simulink model "harm_comp"  (R2020a)
settings: Solver=VariableStepAuto  StartTime=0.0  StopTime=10.0  RelTol=1e-3
values from neighbouring files (symbols this model uses):
  B13 = -params.lmda_f_dc    [run_harmonic_compensation.m]
  comp_table1 = [comp_table1; real(vecs(1,:)*diag(vals)*inv_vecs)]    [run_harmonic_compensation.m]
  Kd0 = [1722.92514708863,-0.149487775533096,     -243.708496078677,0;     0.158174537169950,1528.50661836498,     0,-216.219080907873]    [run_harmonic_compensation.m]
  max_predq = .15    (= 0.15)    [run_harmonic_compensation.m]
  P = params.Poles    [run_harmonic_compensation.m]
  ss_d = H(2,2)    [run_harmonic_compensation.m]
  ss_q = H(1,1)    [run_harmonic_compensation.m]
  start_comp = 50    [run_harmonic_compensation.m]
undefined symbols (not defined in the file or in its folder): baseFreq, T_sw, Vd
settings Model: Creator=adamh  LastModifiedBy=adamh

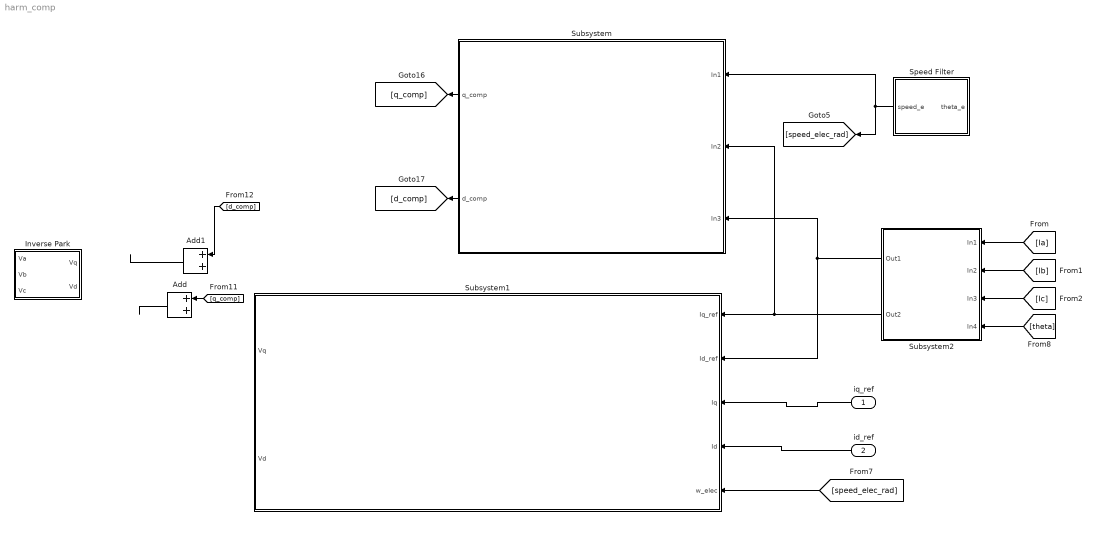
== system harm_comp ==
  iq_ref : Inport
  id_ref : Inport  Port=2
  Add : Sum
  Add1 : Sum
  Inverse Park : Subsystem
  Speed Filter : Subsystem
  Subsystem : Subsystem
      mask Display: image('C:\Users\adamh\Google Drive\AAA Jestie DMD HARMONIC\New_images\Comp_mask.png'); % Use "Edit Image" on toolstrip to change.
  Subsystem1 : Subsystem
      mask Display: image('C:\Users\adamh\Google Drive\AAA Jestie DMD HARMONIC\New_images\Nominal_mask.png'); % Use "Edit Image" on toolstrip to change.
  Subsystem2 : Subsystem
  wires:
  [q_comp] -> Add/1
  [d_comp] -> Add1/1
  Speed Filter/1(speed_e) -> Subsystem/1(In1), [speed_elec_rad]
  Subsystem/1(q_comp) -> [q_comp]
  Subsystem/2(d_comp) -> [d_comp]
  Add1/1 -> ?
  Add/1 -> ?
  iq_ref/1 -> Subsystem1/3("Iq ")
  id_ref/1 -> Subsystem1/4(Id)
  [speed_elec_rad] -> Subsystem1/5(w_elec)
  Subsystem2/2(Out2) -> Subsystem/2(In2), Subsystem1/1(Iq_ref)
  Subsystem2/1(Out1) -> Subsystem1/2(Id_ref), Subsystem/3(In3)
  [Ia] -> Subsystem2/1(In1)
  [Ib] -> Subsystem2/2(In2)
  [Ic] -> Subsystem2/3(In3)
  [theta] -> Subsystem2/4(In4)

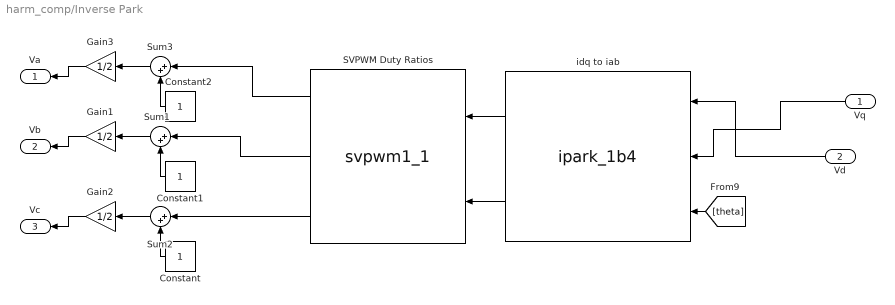
== system harm_comp/Inverse Park ==
  Vq : Inport
  Vd : Inport  Port=2
  Constant : Constant
  Constant1 : Constant
  Constant2 : Constant
  Gain1 : Gain  Gain=1/2
  Gain2 : Gain  Gain=1/2
  Gain3 : Gain  Gain=1/2
  SVPWM Duty Ratios : S-Function  InitFcn=try, set_param(gcb,'FunctionName','svpwm1_1'), end  FunctionName=svpwm1_1  SFunctionModules=svpwm1_1_wrapper  SFunctionDeploymentMode=off  EnableBusSupport=off  mask(S-Function Builder){}
      mask help: Simulink:masks:SFunctionBuilder_MD
      mask init:
      | val = [[.9  0.75 0.75 1 1 .9 .9 1]',[1 1 0.75 0.75 .9 .9 1 .9]'];try , sys = get_param(gcb,'SfunBuilderFcnName');if isempty(sys), sys = get_param(gcb,'FunctionName'); end,catch, sys = get_param(gcb,'FunctionName'); end
      settings: CopyFcn=set_param(gcbh,'LinkStatus','none')  PreSaveFcn=try, set_param(gcb,'FunctionName','svpwm1_1'), end  OpenFcn=sfunctionwizard(gcbh)
      mask Display: plot(val(:,1),val(:,2)),disp(sys), port_label('input',1,'i_alpha'), port_label('input',2,'i_beta'), port_label('output',1,'Ta'), port_label('output',2,'Tb'), port_label('output',3,'Tc')
  Sum1 : Sum  Inputs=|++
  Sum2 : Sum  Inputs=|++
  Sum3 : Sum  Inputs=|++
  idq to iab : S-Function  InitFcn=try, set_param(gcb,'FunctionName','ipark_1b4'), end  FunctionName=ipark_1b4  SFunctionModules=ipark_1b4_wrapper  SFunctionDeploymentMode=off  EnableBusSupport=off  mask(S-Function Builder){}
      mask help: Simulink:masks:SFunctionBuilder_MD
      mask init: same as harm_comp/Inverse Park/SVPWM Duty Ratios
      settings: CopyFcn=set_param(gcbh,'LinkStatus','none')  PreSaveFcn=try, set_param(gcb,'FunctionName','ipark_1b4'), end  OpenFcn=sfunctionwizard(gcbh)
      mask Display: plot(val(:,1),val(:,2)),disp(sys), port_label('input',1,'id'), port_label('input',2,'iq'), port_label('input',3,'theta'), port_label('output',1,'i_alpha'), port_label('output',2,'i_beta')
  Va : Outport
  Vb : Outport  Port=2
  Vc : Outport  Port=3
  wires:
  Sum1/1 -> Gain1/1
  SVPWM Duty Ratios/3 -> Sum2/1
  Sum2/1 -> Gain2/1
  Constant/1 -> Sum2/2
  idq to iab/1 -> SVPWM Duty Ratios/1
  Constant1/1 -> Sum1/2
  SVPWM Duty Ratios/1 -> Sum3/1
  Sum3/1 -> Gain3/1
  idq to iab/2 -> SVPWM Duty Ratios/2
  Gain2/1 -> Vc/1
  [theta] -> idq to iab/3
  SVPWM Duty Ratios/2 -> Sum1/1
  Constant2/1 -> Sum3/2
  Vq/1 -> idq to iab/2
  Vd/1 -> idq to iab/1
  Gain1/1 -> Vb/1
  Gain3/1 -> Va/1

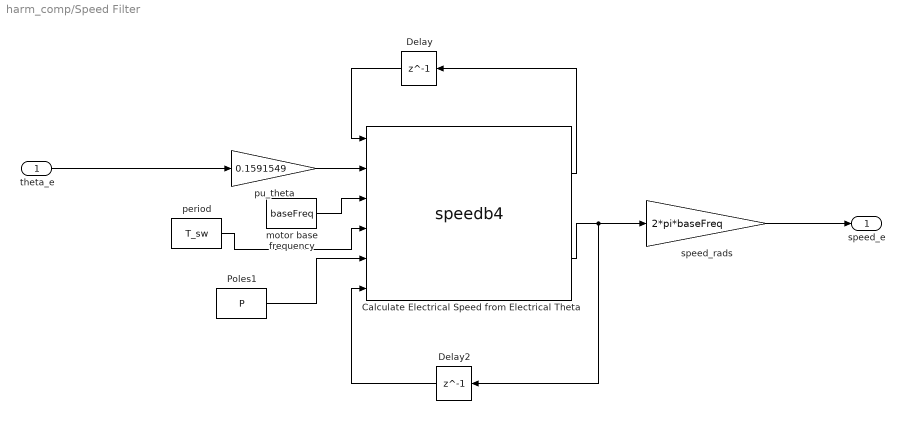
== system harm_comp/Speed Filter ==
  theta_e : Inport
  Calculate Electrical Speed from Electrical Theta : S-Function  InitFcn=try, set_param(gcb,'FunctionName','speedb4'), end  FunctionName=speedb4  SFunctionModules=speedb4_wrapper  SFunctionDeploymentMode=off  EnableBusSupport=off  mask(S-Function Builder){}
      mask help: Simulink:masks:SFunctionBuilder_MD
      mask init: same as harm_comp/Inverse Park/SVPWM Duty Ratios
      settings: CopyFcn=set_param(gcbh,'LinkStatus','none')  PreSaveFcn=try, set_param(gcb,'FunctionName','speedb4'), end  OpenFcn=sfunctionwizard(gcbh)
      mask Display: plot(val(:,1),val(:,2)),disp(sys), port_label('input',1,'oldTheta_in'), port_label('input',2,'theta_in'), port_label('input',3,'baseFreq_in'), port_label('input',4,'T_in'), port_label('input',5,'P_in'), port_label('input',6,'speed_in'), port_label('output',1,'theta_pu'), port_label('output',2,'speed_pu')
  Delay : Delay  DelayLength=1  InitialCondition=0  UseCircularBuffer=on
  Delay2 : Delay  DelayLength=1  InitialCondition=0  UseCircularBuffer=on
  Poles1 : Constant  Value=P
  motor base frequency : Constant  Value=baseFreq
  period : Constant  Value=T_sw
  pu_theta : Gain  Gain=0.1591549
  speed_rads : Gain  Gain=2*pi*baseFreq
  speed_e : Outport
  wires:
  Delay/1 -> Calculate Electrical Speed from Electrical Theta/1
  motor base frequency/1 -> Calculate Electrical Speed from Electrical Theta/3
  Calculate Electrical Speed from Electrical Theta/2 -> speed_rads/1, Delay2/1
  Calculate Electrical Speed from Electrical Theta/1 -> Delay/1
  Poles1/1 -> Calculate Electrical Speed from Electrical Theta/5
  period/1 -> Calculate Electrical Speed from Electrical Theta/4
  pu_theta/1 -> Calculate Electrical Speed from Electrical Theta/2
  Delay2/1 -> Calculate Electrical Speed from Electrical Theta/6
  speed_rads/1 -> speed_e/1
  theta_e/1 -> pu_theta/1

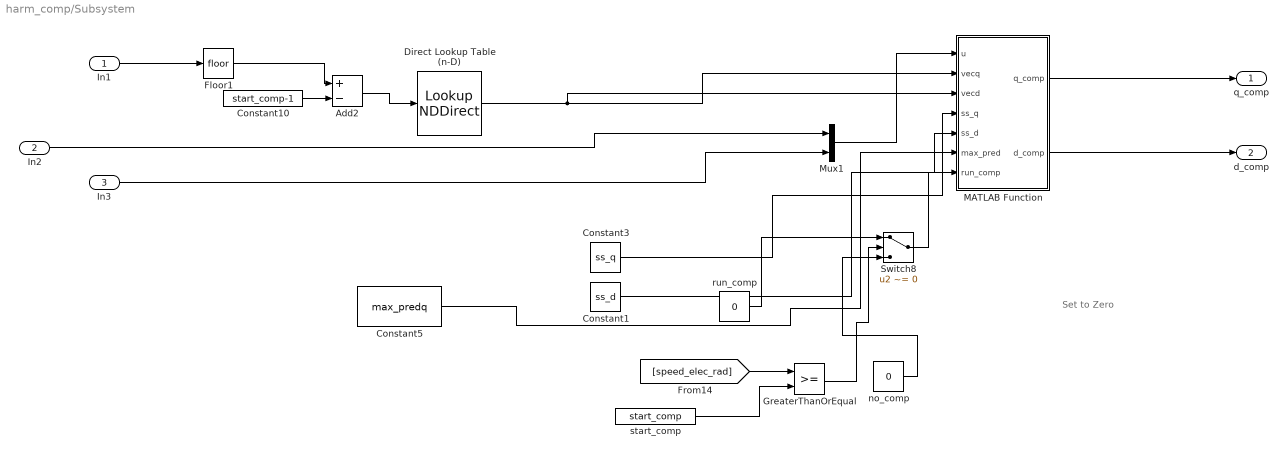
== system harm_comp/Subsystem ==
  note: Set to Zero
  In1 : Inport
  In2 : Inport  Port=2
  In3 : Inport  Port=3
  Add2 : Sum  Inputs=+-
  Constant1 : Constant  Value=ss_d
  Constant10 : Constant  Value=start_comp-1
  Constant3 : Constant  Value=ss_q
  Constant5 : Constant  Value=max_predq
  Direct Lookup Table (n-D) : LookupNDDirect  InputsSelectThisObjectFromTable=Vector  Table=comp_table1'
  Floor1 : Rounding
  GreaterThanOrEqual : RelationalOperator  OutDataTypeStr=boolean  RndMeth=Simplest
  MATLAB Function : MATLAB Function  TreatAsAtomicUnit=on
  Mux1 : Mux  Inputs=2
  Switch8 : Switch  Criteria=u2 ~= 0
  no_comp : Constant  Value=0
  run_comp : Constant  Value=0
  start_comp : Constant  Value=start_comp
  q_comp : Outport
  d_comp : Outport  Port=2
  wires:
  GreaterThanOrEqual/1 -> Switch8/2
  Mux1/1 -> MATLAB Function/1(u)
  no_comp/1 -> Switch8/3
  Constant1/1 -> MATLAB Function/5(ss_d)
  Constant3/1 -> MATLAB Function/4(ss_q)
  Floor1/1 -> Add2/1
  Add2/1 -> Direct Lookup Table (n-D)/1
  Constant5/1 -> MATLAB Function/6(max_pred)
  Direct Lookup Table (n-D)/1 -> MATLAB Function/3(vecd), MATLAB Function/2(vecq)
  start_comp/1 -> GreaterThanOrEqual/2
  [speed_elec_rad] -> GreaterThanOrEqual/1
  Constant10/1 -> Add2/2
  Switch8/1 -> MATLAB Function/7(run_comp)
  run_comp/1 -> Switch8/1
  MATLAB Function/2(d_comp) -> d_comp/1
  In1/1 -> Floor1/1
  MATLAB Function/1(q_comp) -> q_comp/1
  In2/1 -> Mux1/1
  In3/1 -> Mux1/2

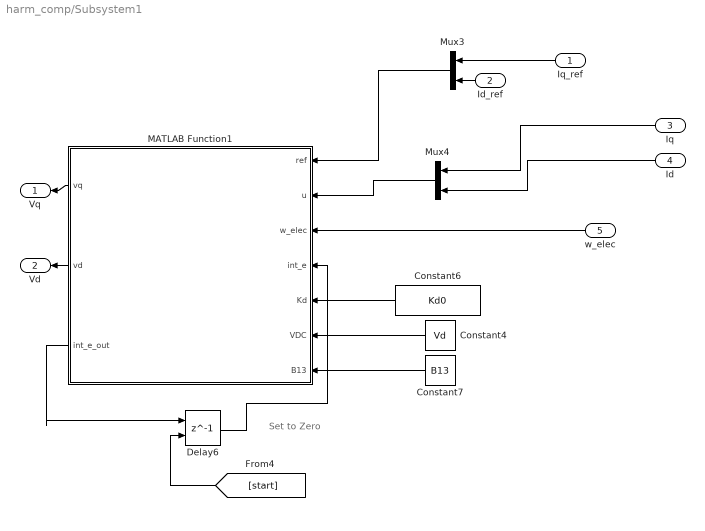
== system harm_comp/Subsystem1 ==
  note: Set to Zero
  Iq_ref : Inport
  Id_ref : Inport  Port=2
  "Iq " : Inport  Port=3
  Id : Inport  Port=4
  w_elec : Inport  Port=5
  Constant4 : Constant  Value=Vd
  Constant6 : Constant  Value=Kd0
  Constant7 : Constant  Value=B13
  Delay6 : Delay  DelayLength=1  ExternalReset=Rising
      settings: InputPortMap=u0,r5
  MATLAB Function1 : MATLAB Function  TreatAsAtomicUnit=on
  Mux3 : Mux  Inputs=2
  Mux4 : Mux  Inputs=2
  Vq : Outport
  Vd : Outport  Port=2
  wires:
  Delay6/1 -> MATLAB Function1/4(int_e)
  MATLAB Function1/3(int_e_out) -> Delay6/1
  Constant7/1 -> MATLAB Function1/7(B13)
  MATLAB Function1/1(vq) -> Vq/1
  Mux4/1 -> MATLAB Function1/2(u)
  Constant4/1 -> MATLAB Function1/6(VDC)
  Mux3/1 -> MATLAB Function1/1(ref)
  Constant6/1 -> MATLAB Function1/5(Kd)
  [start] -> Delay6/2
  Iq_ref/1 -> Mux3/1
  MATLAB Function1/2(vd) -> Vd/1
  Id_ref/1 -> Mux3/2
  "Iq "/1 -> Mux4/1
  w_elec/1 -> MATLAB Function1/3(w_elec)
  Id/1 -> Mux4/2

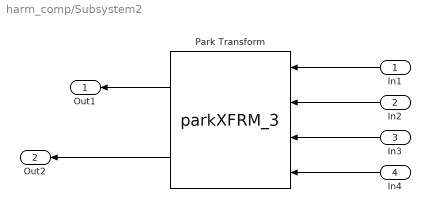
== system harm_comp/Subsystem2 ==
  In1 : Inport
  In2 : Inport  Port=2
  In3 : Inport  Port=3
  In4 : Inport  Port=4
  Park Transform : S-Function  InitFcn=try, set_param(gcb,'FunctionName','parkXFRM_3'), end  FunctionName=parkXFRM_3  SFunctionModules=parkXFRM_3_wrapper  SFunctionDeploymentMode=off  EnableBusSupport=off  mask(S-Function Builder){}
      mask help: Simulink:masks:SFunctionBuilder_MD
      mask init: same as harm_comp/Inverse Park/SVPWM Duty Ratios
      settings: CopyFcn=set_param(gcbh,'LinkStatus','none')  PreSaveFcn=try, set_param(gcb,'FunctionName','parkXFRM_3'), end  OpenFcn=sfunctionwizard(gcbh)
      mask Display: plot(val(:,1),val(:,2)),disp(sys), port_label('input',1,'fa'), port_label('input',2,'fb'), port_label('input',3,'fc'), port_label('input',4,'theta'), port_label('output',1,'fd'), port_label('output',2,'fq')
  Out1 : Outport
  Out2 : Outport  Port=2
  wires:
  In1/1 -> Park Transform/1
  Park Transform/1 -> Out1/1
  Park Transform/2 -> Out2/1
  In2/1 -> Park Transform/2
  In4/1 -> Park Transform/4
  In3/1 -> Park Transform/3

== matlab function harm_comp/Subsystem1/MATLAB Function1 ==
  data: ref input; u input; w_elec input; int_e input; vq output; vd output; int_e_out output; Kd input; VDC input; B13 input
function [vq, vd, int_e_out] = fcn(ref,u,w_elec,int_e, Kd, VDC, B13)

% VDC = 42;

% from Real Parameters
% Ke =[1.6894   -0.1842    0.0000    0.3627   -1.7799    0.3569;
%     0.1842    1.6894   -0.3627    0.0000   -0.3569   -1.7799] ; 
% from fbedmdc
% Ke =[ 2.3940   -0.1699   -0.0016    0.5049   -2.5070    0.2027;
%     0.0938    2.4391   -0.5046   -0.0009   -0.1301   -2.5545];



e = ref - u;
int_e = int_e + e;
% int_e = int_e +Tsd2*e + Tsd2*old_e_in
Kd(1,2) = Kd(1,2)*w_elec;
% Ke(1,4) = Ke(1,4)*w_elec;
Kd(2,1) = Kd(2,1)*w_elec;
% Ke(2,3) = Ke(2,3)*w_elec;


% states = [u(1);u(2);u(1)*factor; u(2)*factor; int_e(1); int_e(2)];
states = [u(1);u(2); int_e(1); int_e(2)];
y = -Kd*states;
y(1) = y(1) - B13*w_elec; % is B13 negative, should be
vq = max(min(y(1), VDC),-VDC);
vd = max(min(y(2), VDC),-VDC);

% vq = vq/VDC;
% vd =vd/VDC;

% vq = y(1)/VDC;
% vd = y(2)/VDC;


int_e_out = int_e;
% old_e = e;
% prevent integrator windup
% if vq ~= y(1) || vd ~= y(2)
%     %satureted
%     int_e_out = int_e - e;
% else
%     int_e_out = int_e;
% end

== matlab function harm_comp/Subsystem/MATLAB Function ==
  data: u input; q_comp output; vecq input; vecd input; ss_q input; ss_d input; max_pred input; run_comp input; d_comp output
function [q_comp, d_comp]  = fcn(u,vecq,vecd, ss_q,ss_d, max_pred, run_comp)

    persistent delayq
    persistent q_pred
    persistent delayd
    persistent d_pred
    
    if isempty(delayq)  
        nEq = length(vecq);
        delayq = zeros(nEq,1);
    end
    if isempty(q_pred)  
        q_pred = 0;
    end
     if isempty(delayd)  
        nEd = length(vecd);
        delayd = zeros(nEd,1);
    end
    if isempty(d_pred)  
        d_pred = 0;
    end  

    
    % compensation
    %protection
    if abs(q_pred)>max_pred || run_comp == 0         
       delayq = [u(1);delayq(1:end-1)]; 
       q_pred = dot(vecq,delayq);
       q_comp=0;
    else

        delayq = [u(1)+q_pred;delayq(1:end-1)];
        q_pred = dot(vecq,delayq); % extract 
        q_comp = ss_q*q_pred;  
    end
    
    if abs(d_pred)>max_pred || run_comp == 0         
       delayd = [u(2);delayd(1:end-1)]; 
       d_pred = dot(vecd,delayd);
       d_comp=0;
    else
        delayd = [u(2)+d_pred;delayd(1:end-1)];
        d_pred = dot(vecd,delayd); % extract 
        d_comp = ss_d*d_pred; 
    end
